simulink model "Comparativa_dinamica_ampliado_complejo_di_puro"  (Simulink 8.3)
settings: Solver=ode45  StartTime=0.0  StopTime=5.0  MaxStep=0.001  RelTol=1e-3
values from neighbouring files (symbols this model uses):
  A = [0 -21.3;0 0]    [DI_implementacion_gacker.m]
  B = [0;-21.3]    [DI_implementacion_gacker.m]
  Cs = eye(size(A,2))    [DI_implementacion_gacker.m]
  Ds = zeros(size(A,2),1)    [DI_implementacion_gacker.m]
  h = 0.05    [DI_implementacion_gacker.m]
  K = double(k)    [DI_implementacion_gacker.m]
  Ka = place(double(pha),double(gma),exp([re+im*i re-im*i pa]*h))    [DI_implementacion_gacker.m]
  tauc = double(tau(2))    [DI_implementacion_gacker.m]
  tauf = 0.03    [DI_implementacion_gacker.m]
settings Model: Creator=mvelasco  LastModifiedBy=mvelasco
settings DataIOCC: SignalLoggingSaveFormat=Dataset
settings DebuggingCC: UnderspecifiedInitializationDetection=Simplified  StateNameClashWarn=none
settings GRTTargetCC: CombineOutputUpdateFcns=on  GRTInterface=off

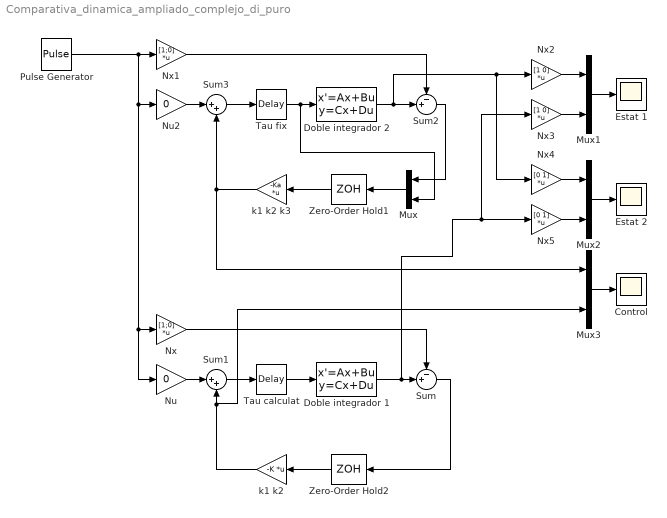
== system Comparativa_dinamica_ampliado_complejo_di_puro ==
  Control : Scope
      settings: SaveName=ScopeData2
  Doble integrador 1 : StateSpace  A=A  B=B  C=Cs  D=Ds  X0=0
  Doble integrador 2 : StateSpace  A=A  B=B  C=Cs  D=Ds  X0=0
  Estat 1 : Scope
      settings: SaveName=estado1
  Estat 2 : Scope
  Mux{,1..3} (4 alike) : Mux  Inputs=2
  Nu : Gain  Gain=0
  Nu2 : Gain  Gain=0
  Nx : Gain  Gain=[1;0]  Multiplication=Matrix(K*u)
  Nx1 : Gain  Gain=[1;0]  Multiplication=Matrix(K*u)
  Nx2 : Gain  Gain=[1 0]  Multiplication=Matrix(K*u)
  Nx3 : Gain  Gain=[1 0]  Multiplication=Matrix(K*u)
  Nx4 : Gain  Gain=[0 1]  Multiplication=Matrix(K*u)
  Nx5 : Gain  Gain=[0 1]  Multiplication=Matrix(K*u)
  Pulse Generator : DiscretePulseGenerator  PulseType=Time based  PulseWidth=50
  Sum : Sum  Inputs=-+|
  Sum1 : Sum  Inputs=|++
  Sum2 : Sum  Inputs=-+|
  Sum3 : Sum  Inputs=|++
  Tau calculat : TransportDelay  DelayTime=tauc
  Tau fix : TransportDelay  DelayTime=tauf
  Zero-Order Hold1 : ZeroOrderHold  SampleTime=h
  Zero-Order Hold2 : ZeroOrderHold  SampleTime=h
  k1 k2 : Gain  Gain=-K  Multiplication=Matrix(K*u)
  k1 k2 k3 : Gain  Gain=-Ka  Multiplication=Matrix(K*u)
  wires:
  Pulse Generator/1 -> Nu/1, Nx/1, Nu2/1, Nx1/1
  Nx/1 -> Sum/1
  Doble integrador 1/1 -> Nx3/1, Nx5/1, Sum/2
  Sum/1 -> Zero-Order Hold2/1
  k1 k2/1 -> Mux3/2, Sum1/2
  Nu/1 -> Sum1/1
  Sum1/1 -> Tau calculat/1
  Tau calculat/1 -> Doble integrador 1/1
  Zero-Order Hold2/1 -> k1 k2/1
  Nx1/1 -> Sum2/1
  Doble integrador 2/1 -> Nx4/1, Nx2/1, Sum2/2
  k1 k2 k3/1 -> Mux3/1, Sum3/2
  Nu2/1 -> Sum3/1
  Sum3/1 -> Tau fix/1
  Tau fix/1 -> Mux/2, Doble integrador 2/1
  Zero-Order Hold1/1 -> k1 k2 k3/1
  Mux/1 -> Zero-Order Hold1/1
  Sum2/1 -> Mux/1
  Mux1/1 -> Estat 1/1
  Nx2/1 -> Mux1/1
  Nx3/1 -> Mux1/2
  Mux2/1 -> Estat 2/1
  Nx4/1 -> Mux2/1
  Nx5/1 -> Mux2/2
  Mux3/1 -> Control/1
